simulink model "PV_Systerm_loser"  (R2025b)
settings: Solver=VariableStepAuto  StartTime=0.0  StopTime=0.2  RelTol=1e-3
undefined symbols (not defined in the file or in its folder): Down, Up
libraries: fl_lib x7, nesl_utility x5, ee_lib x2, eePwmGenerator x1
settings Model: Creator=19816  LastModifiedBy=19816
settings SolverCC: ZeroCrossAlgorithm=Adaptive
settings DebuggingCC: AlgebraicLoopMsg=none  MaskedZcDiagnostic=none  IgnoredZcDiagnostic=none

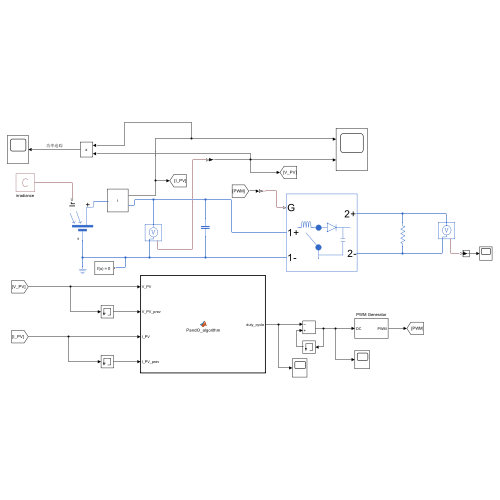
[thumbnail: Simulink's stored preview of the top-level diagram]
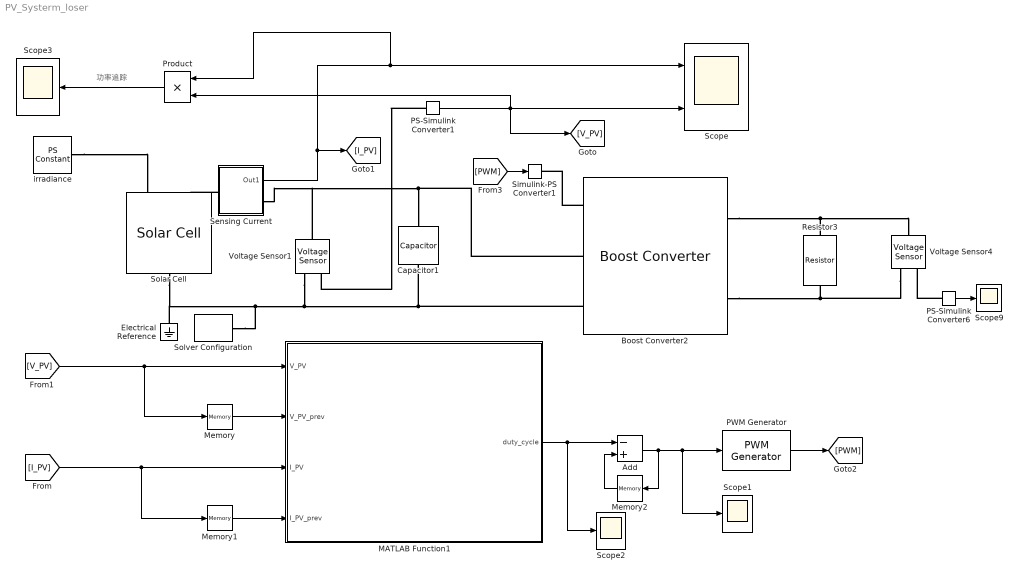
== system PV_Systerm_loser ==
  note: 功率追踪
  Add : Sum  Inputs=-+
  Boost Converter2 : ee_lib/Semiconductors & Converters/Converters/Boost Converter  port_option=ee.enum.controlport.ps  device_type=ee.enum.converters.switchingdevice.igbt  Vf=0.8 V  Ron=0.001 Ohm  Rds=0.001 Ohm  Goff=1e-5 1/Ohm  Vgt=1 V  Vgt_off=-1 V  Ih=1 A  Vth=0.5 V  K=0  diode_param=ee.enum.converters.protectiondiode.nodynamics  diode_Vf=0.8 V  diode_Ron=0.001 Ohm  diode_Goff=1e-5 1/Ohm  diode_C=50 nF  diode_iRM=-235 A  diode_iF=300 A  diode_idot=-50 A/us  diode_trr_param=ee.enum.converters.diodetrr.trr_factor  diode_trr_factor=3  diode_trr=15 us  diode_Qrr=1500 s*uA  Lf=1e-2 H  Rl=0 Ohm  Cf=1e-2 F  Rf=1e-6 Ohm  snubber_type=ee.enum.converters.snubber.exclude  Cs=1e-7 F  Rs=0.1 Ohm  iL_specify=off  iL_priority=High  iL=0 A  iL_nominal_specify=off  iL_nominal_value=1  iL_nominal_unit=A  vc_specify=off  vc_priority=High  vc=0 V  vc_nominal_specify=off  vc_nominal_value=1  vc_nominal_unit=V
      settings: InternalSimscapePortConfiguration="{\"Bottom\":[],\"Left\":[{\"id\":\"G\",\"label\":\"G\",\"type\":\"input\"},{\"id\":\"p1\",\"label\":\"1+\",\"type\":\"foundation.electrical.electrical\"},{\"id\":\"n1\",\"label\":\"1-\",\"type\":\"foundation.electrical.electrical\"}],\"Right\":[{\"id\":\"p2\",\"label\":\"2+\",\"type\":\"foundation.electrical.electrical\"},{\"id\":\"n2\",\"label\":\"2-\",\"type\":\"foundation.electrical.electrical\"}],\"Top\":[]}"
  Capacitor1 : fl_lib/Electrical/Electrical Elements/Capacitor  c=1e-3 F  r=1e-6 Ohm  g=0 1/Ohm  i_specify=off  i_priority=None  i=0 A  i_nominal_specify=off  i_nominal_value=1  i_nominal_unit=A  v_specify=off  v_priority=None  v=0 V  v_nominal_specify=off  v_nominal_value=1  v_nominal_unit=V  vc_specify=off  vc_priority=High  vc=0 V  vc_nominal_specify=off  vc_nominal_value=1  vc_nominal_unit=V
  Electrical Reference : fl_lib/Electrical/Electrical Elements/Electrical Reference
  MATLAB Function1 : MATLAB Function  TreatAsAtomicUnit=on
  Memory : Memory
  Memory1 : Memory
  Memory2 : Memory
  PS-Simulink Converter1 : nesl_utility/PS-Simulink Converter  PhysicalDomain=network_engine_domain  SubClassName=ps_output  LeftPortType=input  RightPortType=output  PseudoPeriodic=off  Frequencies=[]  VectorFormat=inherit  Unit=inherit  AffineConversion=off
  PS-Simulink Converter6 : nesl_utility/PS-Simulink Converter  PhysicalDomain=network_engine_domain  SubClassName=ps_output  LeftPortType=input  RightPortType=output  PseudoPeriodic=off  Frequencies=[]  VectorFormat=inherit  Unit=inherit  AffineConversion=off
  PWM Generator : eePwmGenerator/PWM Generator  CarrCount=Up-Down  Tper=0.0001  Tdelay=0  Ts=0
  Product : Product
  Resistor3 : fl_lib/Electrical/Electrical Elements/Resistor  R=0.912 Ohm  i_specify=off  i_priority=None  i=0 A  i_nominal_specify=off  i_nominal_value=1  i_nominal_unit=A  v_specify=off  v_priority=None  v=0 V  v_nominal_specify=off  v_nominal_value=1  v_nominal_unit=V
  Scope : Scope  NumInputPorts=2
      settings: ActiveDisplayYMinimum=1.7672323036405242  ActiveDisplayYMaximum=13.579343171550992  DataLoggingVariableName=ScopeData2
  Scope{1..3,9} (4 alike) : Scope
      Scope1 settings: ActiveDisplayYMinimum=-0.97617690552607517  ActiveDisplayYMaximum=1.4698129710132131  DataLoggingVariableName=ScopeData3
      Scope2 settings: ActiveDisplayYMinimum=-0.97617690552607517  ActiveDisplayYMaximum=1.4698129710132131
      Scope3 settings: ActiveDisplayYMinimum=552.08230671387321  ActiveDisplayYMaximum=1155.4900322573112
      Scope9 settings: ActiveDisplayYMinimum=-2.1924635461181694  ActiveDisplayYMaximum=89.977855479510993  DataLoggingVariableName=ScopeData9
  Sensing Current : Subsystem
      mask Display: disp('i')
  Simulink-PS Converter1 : nesl_utility/Simulink-PS Converter  PhysicalDomain=network_engine_domain  SubClassName=ps_input  LeftPortType=input  RightPortType=output  PseudoPeriodic=off  Frequencies=[]  NoiseDistribution=none  NoiseParameters=[]  Unit=1  AffineConversion=off  FilteringAndDerivatives=provide  SimscapeFilterOrder=1  InputFilterTimeConstant=0.001  UdotUserProvided=0
  Solar Cell : ee_lib/Sources/Solar Cell  prm=ee.enum.sources.solar_cell_prm.datasheet  Isc=7.34 A  Voc=0.6 V  Is=1e-6 A  Is2=0 A  Iph=7.34 A  Ir0=1000 W/m^2  ec=1.5  N2=2  Rs=0 Ohm  Rp=inf Ohm  N_series=60  N_parallel=5  TIPH1=0 1/K  EG=1.11 eV  TXIS1=3  TXIS2=3  TRS1=0  TRP1=0  Tmeas=25 degC  TFIXED=25 degC  thermal_mass=100 J/K  initial_temperature=25 degC
  Solver Configuration : nesl_utility/Solver Configuration  PhysicalDomain=network_engine_domain  SubClassName=solver  LeftPortType=input  RightPortType=generic  Tones=[]  Harmonics=[]  SimulateNoise=off  Profile=off  UseLocalSampling=off  EnableSwitchedLinearOptims=on  FrequencyDomain=off  UseCCode=off  RelTol=0.001  AbsTol=0.001  MinStep=1e-09  ToWorkspace=off  RevertToSquareIcSolve=off  NumHomotopyIterations=100  PhasorMode=off  PhasorModeNumHarmonics=1  ConsistencySolver=NEWTON_XTOL_AFTER_FTOL  IndexReductionMethod=DerivativeReplacement  DoDC=off  ResidualTolerance=1e-09  ConsistencyTolSource=GLOBAL  ConsistencyAbsTol=0.001  ConsistencyRelTol=0.001  ConsistencyTolFactor=0.001  UseLocalSolver=off  LocalSolverChoice=NE_BACKWARD_EULER_ADVANCER  ResolveIndetEquations=on  FunctionEvalNumThread=1  LocalSolverSampleTime=0.001  DoFixedCost=off  MaxNonlinIter=3  MaxModeIter=2  ComputeImpulses=off  ImpulseIterations=2  LinearAlgebra=auto  LinearAlgebraNumThread=0  EquationFormulation=NE_TIME_EF  DelaysMemoryBudget=1024  AutomaticFiltering=on  FilteringTimeConstant=0.001  PartitionStorageMethod=AS_NEEDED  PartitionMemoryBudget=1024  PartitionMethod=ROBUST  MultibodyUseLocalSolver=off  MultibodyLocalSolverChoice=ODE1  MultibodyLocalSolverSampleTime=0.001
  Voltage Sensor1 : fl_lib/Electrical/Electrical Sensors/Voltage Sensor
  Voltage Sensor4 : fl_lib/Electrical/Electrical Sensors/Voltage Sensor
  irradiance : fl_lib/Physical Signals/Sources/PS Constant  constant=1000
  wires:
  [I_PV] -> Memory1/1, MATLAB Function1/3(I_PV)
  [V_PV] -> Memory/1, MATLAB Function1/1(V_PV)
  Memory/1 -> MATLAB Function1/2(V_PV_prev)
  Memory1/1 -> MATLAB Function1/4(I_PV_prev)
  Product/1 -> Scope3/1
  Sensing Current/1(Out1) -> Product/1, Scope/1, [I_PV]
  PS-Simulink Converter1/1 -> Product/2, [V_PV], Scope/2
  Add/1 -> Scope1/1, PWM Generator/1, Memory2/1
  PWM Generator/1 -> [PWM]
  PS-Simulink Converter6/1 -> Scope9/1
  [PWM] -> Simulink-PS Converter1/1
  MATLAB Function1/1(duty_cycle) -> Scope2/1, Add/1
  Memory2/1 -> Add/2
  connections:
  Solver Configuration/RConn1 -- Electrical Reference/LConn1 -- Solar Cell/RConn1 -- Voltage Sensor1/RConn2 -- Capacitor1/RConn1 -- Boost Converter2/LConn3
  Voltage Sensor1/LConn1 -- Sensing Current/RConn1 -- Boost Converter2/LConn2 -- Capacitor1/LConn1
  irradiance/RConn1 -- Solar Cell/LConn1
  Sensing Current/LConn1 -- Solar Cell/LConn2
  PS-Simulink Converter1/LConn1 -- Voltage Sensor1/RConn1
  Boost Converter2/RConn1 -- Resistor3/RConn1 -- Voltage Sensor4/LConn1
  Boost Converter2/RConn2 -- Voltage Sensor4/RConn2 -- Resistor3/LConn1
  PS-Simulink Converter6/LConn1 -- Voltage Sensor4/RConn1
  Boost Converter2/LConn1 -- Simulink-PS Converter1/RConn1

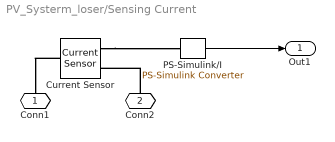
== system PV_Systerm_loser/Sensing Current ==
  Current Sensor : fl_lib/Electrical/Electrical Sensors/Current Sensor
  PS-Simulink/I : nesl_utility/PS-Simulink Converter  PhysicalDomain=network_engine_domain  SubClassName=ps_output  LeftPortType=input  RightPortType=output  PseudoPeriodic=off  Frequencies=[]  VectorFormat=1-D array  Unit=1  AffineConversion=off
  Conn1 : PMIOPort  Side=Left
  Conn2 : PMIOPort  Port=2  Side=Right
  Out1 : Outport  VectorParamsAs1DForOutWhenUnconnected=off
  wires:
  PS-Simulink/I/1 -> Out1/1
  connections:
  Current Sensor/RConn1 -- PS-Simulink/I/LConn1
  Current Sensor/LConn1 -- Conn1/RConn1
  Conn2/RConn1 -- Current Sensor/RConn2

== matlab function PV_Systerm_loser/MATLAB Function1 ==
  data: V_PV input; V_PV_prev input; I_PV input; duty_cycle output; I_PV_prev input
function duty_cycle  = PandO_algorithm(V_PV, V_PV_prev , I_PV, I_PV_prev)
% 扰动观察法I_PV
% 光伏电池参数
k1 = 0.01;
k2 = 0.001;
P_threshold = 55; % 设定阈值
V_threshold = 1; % 设定阈值

P_PV_prev = V_PV_prev * I_PV_prev;
P_PV = V_PV * I_PV;
dP = abs(P_PV - P_PV_prev);
dV = abs(V_PV - V_PV_prev);
sgn = sign(P_PV - P_PV_prev);
    
% 判断功率变化方向
if dP > P_threshold
   step =k1 * dP; % 大功率下步长变大 
elseif dV < V_threshold
   step =k2 * dP; % 接近极值点时缩小步长
else
   step = 0.01; % 默认步长
end

duty_cycle = sgn * step;
end
